simulink model "ex6_model"  (R2013a)
settings: Solver=ode45  StartTime=0.0  StopTime=10.0  RelTol=1e-3
values from neighbouring files (symbols this model uses):
  g = 0.81    [ex6.m]
  k = 1    [ex5.m]    (also in ex6.m = 0.001)
  K = 49    [ex5.m]    (also in ex6.m = 1)
  m = 1    [ex5.m]    (also in ex6.m = 0.1)
  q_0 = 0    [ex6.m]
  q_dot_0 = 0    [ex6.m]
  w = 10    [ex6.m]
settings Model: Creator=Brent  LastModifiedBy=Willdog

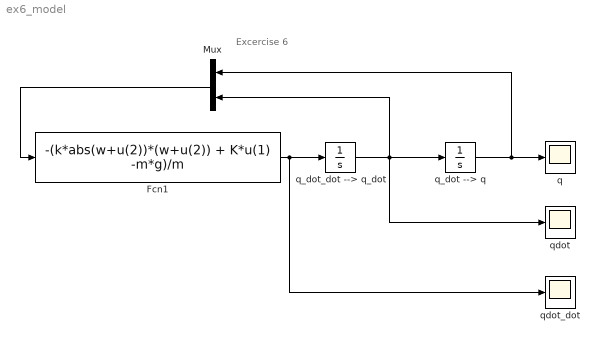
== system ex6_model ==
  note: Excercise 6
  Fcn1 : Fcn  Expr=-(k*abs(w+u(2))*(w+u(2)) + K*u(1) -m*g)/m
  Mux : Mux  Inputs=2
  q : Scope
  q_dot --> q : Integrator  InitialCondition=q_0
  q_dot_dot --> q_dot : Integrator  InitialCondition=q_dot_0
  qdot : Scope
  qdot_dot : Scope
      settings: SaveName=ScopeData2
  wires:
  q_dot_dot --> q_dot/1 -> qdot/1, Mux/2, q_dot --> q/1
  q_dot --> q/1 -> Mux/1, q/1
  Mux/1 -> Fcn1/1
  Fcn1/1 -> qdot_dot/1, q_dot_dot --> q_dot/1
